simulink model "pi_drive"  (R2019a)
settings: Solver=FixedStepAuto  StartTime=0.0  StopTime=inf  FixedStep=sT  RelTol=1e-3  EnableMultiTasking=on
InitFcn:
  | sT = 0.01;
libraries: raspberrypilib x5
settings Model: SimulationMode=external  Creator=hideaki  LastModifiedBy=hideaki
settings SolverCC: PositivePriorityOrder=on
settings DataIOCC: ReturnWorkspaceOutputs=off
settings OptimizationCC: EnhancedBackFolding=on  PassReuseOutputArgsThreshold=0  MaxStackSize=64  OptimizeBlockOrder=speed  DifferentSizesBufferReuse=on  OptimizationCustomize=off
settings DebuggingCC: ParameterTunabilityLossMsg=error  ArithmeticOperatorsInVariantConditions=warning
settings HardwareCC: ProdBitPerPointer=32  ProdBitPerSizeT=32  ProdBitPerPtrDiffT=32  ProdLargestAtomicInteger=Long  ProdLargestAtomicFloat=Double  ProdWordSize=32  ProdHWDeviceType=ARM Compatible->ARM Cortex  UseEmbeddedCoderFeatures=off  UseSimulinkCoderFeatures=off
settings SFSimCC: MATLABDynamicMemAlloc=off
settings RTWCC: SystemTargetFile=ert.tlc  HardwareBoard=Raspberry Pi  TLCOptions="-aInlineSetEventsForThisBaseRateFcn=TLC_FALSE -aSuppressMultiTaskScheduler=TLC_FALSE  -aRateBasedStepFcn=0"  TemplateMakefile=ert_default_tmf  GenerateReport=on  Toolchain=GNU GCC Raspberry Pi  BuildConfiguration=Faster Runs  LaunchReport=on
settings CodeAppCC: ForceParamTrailComments=on  OperatorAnnotations=on  MangleLength=10
settings ERTTargetCC: TargetLangStandard=C99 (ISO)  ERTCustomFileBanners=off  SupportContinuousTime=on  SupportNonInlinedSFcns=on  RemoveResetFunc=off  SupportVariableSizeSignals=on  ModelStepFunctionPrototypeControlCompliant=off

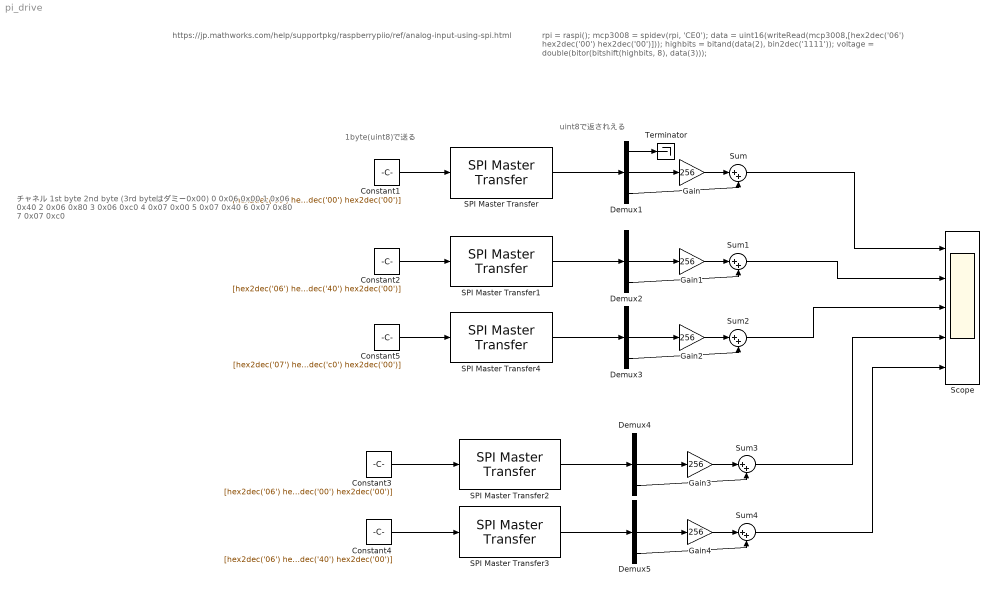
== system pi_drive ==
  note: チャネル 1st byte 2nd byte (3rd byteはダミー0x00)
      | 0 0x06 0x00
      | 1 0x06 0x40
      | 2 0x06 0x80
      | 3 0x06 0xc0
      | 4 0x07 0x00
      | 5 0x07 0x40
      | 6 0x07 0x80
      | 7 0x07 0xc0
  note: uint8で返されえる
  note: 1byte(uint8)で送る
  note: https://jp.mathworks.com/help/supportpkg/raspberrypiio/ref/analog-input-using-spi.html
  note: rpi = raspi();
      | mcp3008 = spidev(rpi, 'CE0');
      | data = uint16(writeRead(mcp3008,[hex2dec('06') hex2dec('00') hex2dec('00')]));
      | highbits = bitand(data(2), bin2dec('1111'));
      | voltage = double(bitor(bitshift(highbits, 8), data(3)));
  Constant1 : Constant  Value=[hex2dec('06') hex2dec('00') hex2dec('00')]  OutDataTypeStr=uint8
  Constant2 : Constant  Value=[hex2dec('06') hex2dec('40') hex2dec('00')]  OutDataTypeStr=uint8
  Constant3 : Constant  Value=[hex2dec('06') hex2dec('00') hex2dec('00')]  OutDataTypeStr=uint8
  Constant4 : Constant  Value=[hex2dec('06') hex2dec('40') hex2dec('00')]  OutDataTypeStr=uint8
  Constant5 : Constant  Value=[hex2dec('07') hex2dec('c0') hex2dec('00')]  OutDataTypeStr=uint8
  Demux{1..5} (5 alike) : Demux  Outputs=3
  Gain{,1..4} (5 alike) : Gain  Gain=256
  SPI Master Transfer : raspberrypilib/SPI Master Transfer  BoardProperty=Pi 3 Model B  SPIModule=uint32(0)  Mode=Master  BusSpeed=1000000  Pin=SPI0_CE0  FirstBitToTransfer=Most significant bit (MSB)  ClockMode=0  BlockFunction=Transfer  RegisterAddress=0  OutputDataType=int8  OutputDataLength=1
      settings: SourceProductName=Simulink Support Package for Raspberry Pi Hardware  SourceProductBaseCode=RASPPI
  SPI Master Transfer1 : raspberrypilib/SPI Master Transfer  BoardProperty=Pi 3 Model B  SPIModule=uint32(0)  Mode=Master  BusSpeed=1000000  Pin=SPI0_CE0  FirstBitToTransfer=Most significant bit (MSB)  ClockMode=0  BlockFunction=Transfer  RegisterAddress=0  OutputDataType=int8  OutputDataLength=1
      settings: SourceProductName=Simulink Support Package for Raspberry Pi Hardware  SourceProductBaseCode=RASPPI
  SPI Master Transfer2 : raspberrypilib/SPI Master Transfer  BoardProperty=Pi 3 Model B  SPIModule=uint32(0)  Mode=Master  BusSpeed=1000000  Pin=SPI0_CE1  FirstBitToTransfer=Most significant bit (MSB)  ClockMode=0  BlockFunction=Transfer  RegisterAddress=0  OutputDataType=int8  OutputDataLength=1
      settings: SourceProductName=Simulink Support Package for Raspberry Pi Hardware  SourceProductBaseCode=RASPPI
  SPI Master Transfer3 : raspberrypilib/SPI Master Transfer  BoardProperty=Pi 3 Model B  SPIModule=uint32(0)  Mode=Master  BusSpeed=1000000  Pin=SPI0_CE1  FirstBitToTransfer=Most significant bit (MSB)  ClockMode=0  BlockFunction=Transfer  RegisterAddress=0  OutputDataType=int8  OutputDataLength=1
      settings: SourceProductName=Simulink Support Package for Raspberry Pi Hardware  SourceProductBaseCode=RASPPI
  SPI Master Transfer4 : raspberrypilib/SPI Master Transfer  BoardProperty=Pi 3 Model B  SPIModule=uint32(0)  Mode=Master  BusSpeed=1000000  Pin=SPI0_CE0  FirstBitToTransfer=Most significant bit (MSB)  ClockMode=0  BlockFunction=Transfer  RegisterAddress=0  OutputDataType=int8  OutputDataLength=1
      settings: SourceProductName=Simulink Support Package for Raspberry Pi Hardware  SourceProductBaseCode=RASPPI
  Scope : Scope  NumInputPorts=5
  Sum{,1..4} (5 alike) : Sum  Inputs=|++
  Terminator : Terminator
  wires:
  Constant1/1 -> SPI Master Transfer/1
  Constant2/1 -> SPI Master Transfer1/1
  Constant3/1 -> SPI Master Transfer2/1
  Constant4/1 -> SPI Master Transfer3/1
  Constant5/1 -> SPI Master Transfer4/1
  SPI Master Transfer/1 -> Demux1/1
  Demux1/2 -> Gain/1
  Demux1/1 -> Terminator/1
  Gain/1 -> Sum/1
  Demux1/3 -> Sum/2
  Sum/1 -> Scope/1
  Sum1/1 -> Scope/2
  Demux2/3 -> Sum1/2
  Gain1/1 -> Sum1/1
  Demux2/2 -> Gain1/1
  SPI Master Transfer1/1 -> Demux2/1
  Sum2/1 -> Scope/3
  Demux3/3 -> Sum2/2
  Gain2/1 -> Sum2/1
  Demux3/2 -> Gain2/1
  SPI Master Transfer4/1 -> Demux3/1
  Demux4/3 -> Sum3/2
  Gain3/1 -> Sum3/1
  Demux4/2 -> Gain3/1
  SPI Master Transfer2/1 -> Demux4/1
  Demux5/3 -> Sum4/2
  Gain4/1 -> Sum4/1
  Demux5/2 -> Gain4/1
  SPI Master Transfer3/1 -> Demux5/1
  Sum3/1 -> Scope/4
  Sum4/1 -> Scope/5
